simulink model "mode_lame_2019b_tentative2"  (R2020b)
settings: Solver=VariableStepAuto  StartTime=0.0  StopTime=10  RelTol=1e-3
settings Model: Creator=antoi  LastModifiedBy=antoi
settings DebuggingCC: UnderSpecifiedDimensionMsg=warning

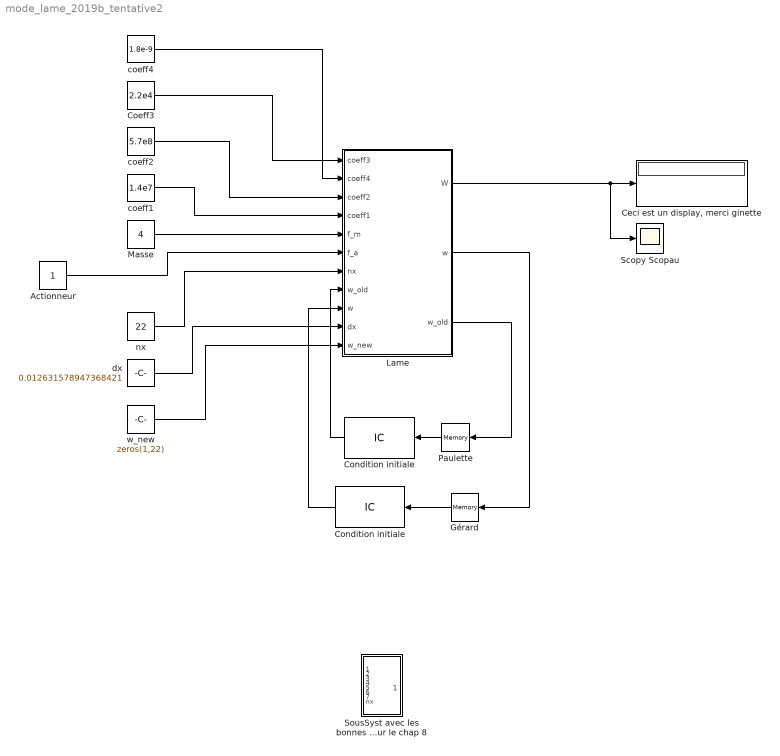
== system mode_lame_2019b_tentative2 ==
  Actionneur : Constant
  "Ceci est un display, merci ginette" : Display
  Coeff3 : Constant  Value=2.2e4
  Condition initiale : InitialCondition  Value=zeros(1,22)
  "Condition initiale " : InitialCondition  Value=zeros(1,22)
  Gérard : Memory
  Lame : MATLAB Function  TreatAsAtomicUnit=on
  Masse : Constant  Value=4
  Paulette : Memory
  Scopy Scopau : Scope
  SousSyst avec les bonnes entrées pour le chap 8 : Subsystem
  coeff1 : Constant  Value=1.4e7
  coeff2 : Constant  Value=5.7e8
  coeff4 : Constant  Value=1.8e-9
  dx : Constant  Value=0.012631578947368421
  nx : Constant  Value=22
  w_new : Constant  Value=zeros(1,22)
  wires:
  Masse/1 -> Lame/5(f_m)
  Lame/2(w) -> Gérard/1
  Lame/3(w_old) -> Paulette/1
  Gérard/1 -> Condition initiale/1
  Paulette/1 -> "Condition initiale "/1
  Lame/1(W) -> Scopy Scopau/1, "Ceci est un display, merci ginette"/1
  Coeff3/1 -> Lame/1(coeff3)
  coeff4/1 -> Lame/2(coeff4)
  nx/1 -> Lame/7(nx)
  "Condition initiale "/1 -> Lame/8("w_old ")
  Condition initiale/1 -> Lame/9("w ")
  coeff2/1 -> Lame/3(coeff2)
  dx/1 -> Lame/10(dx)
  w_new/1 -> Lame/11(w_new)
  Actionneur/1 -> Lame/6(f_a)
  coeff1/1 -> Lame/4(coeff1)

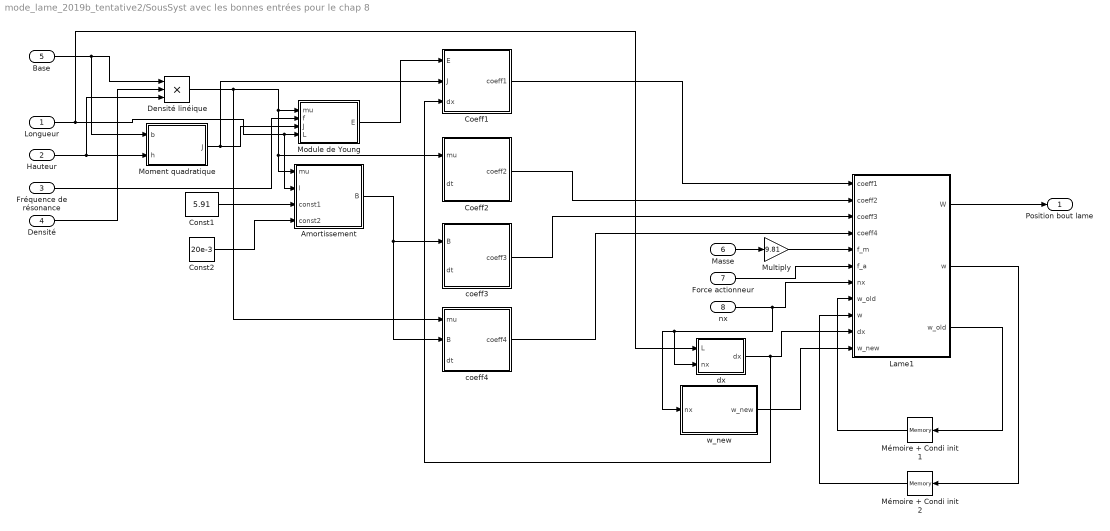
== system mode_lame_2019b_tentative2/SousSyst avec les bonnes entrées pour le chap 8 ==
  Longueur : Inport
  Hauteur : Inport  Port=2
  Fréquence de résonance : Inport  Port=3
  Densité : Inport  Port=4
  Base : Inport  Port=5
  Masse : Inport  Port=6
  Force actionneur : Inport  Port=7
  nx : Inport  Port=8
  Amortissement : MATLAB Function  TreatAsAtomicUnit=on
  Coeff1 : MATLAB Function  TreatAsAtomicUnit=on
  Coeff2 : MATLAB Function  TreatAsAtomicUnit=on
  Const1 : Constant  Value=5.91
  Const2 : Constant  Value=20e-3
  Densité linéique : Product  Inputs=3
  Lame1 : MATLAB Function  TreatAsAtomicUnit=on
  Module de Young : MATLAB Function  TreatAsAtomicUnit=on
  Moment quadratique : MATLAB Function  TreatAsAtomicUnit=on
  Multiply : Gain  Gain=9.81
  Mémoire + Condi init 1 : Memory  InitialCondition=zeros(1,22)
  Mémoire + Condi init 2 : Memory  InitialCondition=zeros(1,22)
  coeff3 : MATLAB Function  TreatAsAtomicUnit=on
  coeff4 : MATLAB Function  TreatAsAtomicUnit=on
  dx : MATLAB Function  TreatAsAtomicUnit=on
  w_new : MATLAB Function  TreatAsAtomicUnit=on
  Position bout lame : Outport
  wires:
  Lame1/3(w_old) -> Mémoire + Condi init 1/1
  Lame1/2(w) -> Mémoire + Condi init 2/1
  Mémoire + Condi init 1/1 -> Lame1/8("w_old ")
  Mémoire + Condi init 2/1 -> Lame1/9("w ")
  Lame1/1(W) -> Position bout lame/1
  Base/1 -> Moment quadratique/1(b), Densité linéique/1
  Densité/1 -> Densité linéique/2
  Hauteur/1 -> Densité linéique/3, Moment quadratique/2(h)
  Densité linéique/1 -> coeff4/1(mu), Coeff2/1(mu), Amortissement/1(mu), Module de Young/1(mu)
  Moment quadratique/1(J) -> Coeff1/2(J), Module de Young/3(J)
  Fréquence de résonance/1 -> Module de Young/2(f)
  Longueur/1 -> dx/1(L), Amortissement/2(l), Module de Young/4(L)
  Const1/1 -> Amortissement/3(const1)
  Const2/1 -> Amortissement/4(const2)
  Coeff1/1(coeff1) -> Lame1/1(coeff1)
  Coeff2/1(coeff2) -> Lame1/2(coeff2)
  coeff3/1(coeff3) -> Lame1/3(coeff3)
  coeff4/1(coeff4) -> Lame1/4(coeff4)
  Masse/1 -> Multiply/1
  Multiply/1 -> Lame1/5(f_m)
  Force actionneur/1 -> Lame1/6(f_a)
  nx/1 -> w_new/1(nx), dx/2(nx), Lame1/7(nx)
  dx/1(dx) -> Coeff1/3(dx), Lame1/10(dx)
  w_new/1(w_new) -> Lame1/11(w_new)
  Module de Young/1(E) -> Coeff1/1(E)
  Amortissement/1(B) -> coeff4/2(B), coeff3/1(B)

== matlab function mode_lame_2019b_tentative2/SousSyst avec les bonnes entrées pour le chap 8/Coeff2 ==
  data: mu input; coeff2 output; dt input
function coeff2 = fcn(mu, dt)

coeff2 = mu/(dt^2);

== matlab function mode_lame_2019b_tentative2/SousSyst avec les bonnes entrées pour le chap 8/Coeff1 ==
  data: E input; coeff1 output; J input; dx input
function coeff1 = fcn(E, J, dx)

coeff1 = (E * J)/(dx^4);

== matlab function mode_lame_2019b_tentative2/SousSyst avec les bonnes entrées pour le chap 8/dx ==
  data: L input; dx output; nx input
function dx = fcn(L, nx)

dx = L/(nx-1);

== matlab function mode_lame_2019b_tentative2/SousSyst avec les bonnes entrées pour le chap 8/w_new ==
  data: w_new output; nx input
function w_new = fcn(nx)

w_new = zeroes(1,nx);

== matlab function mode_lame_2019b_tentative2/SousSyst avec les bonnes entrées pour le chap 8/Lame1 ==
  data: coeff1 input; coeff2 input; coeff3 input; coeff4 input; f_m input; W output; f_a input; nx input; w_old input; w input; dx input; w output; w_old output; w_new input
function [W, w, w_old] = fcn(coeff1, coeff2, coeff3, coeff4, f_m, f_a, nx, w_old, w, dx, w_new) 
    
    % Vecteur position
    %w_new = zeros(1,nx); %PO y dit non non non
    
    
    % La force
    F = zeros(1, nx);
    F(11) = f_a + f_m;
    
    
%     h = plot(x, w_init, x, w_new);
%     xlabel("X [m]")
%     ylabel("Déflexion [m]")
%     ylim([-0.01,0.01])
%     grid on

    
    for i = 3:nx-2
        
        %Équation différentielle résolue par Sam
        w_new(i) = (-coeff1*(w(i+2)-4*w(i+1)+6*w(i)-4*w(i-1)+w(i-2)) - coeff2*(-2*w(i)+w_old(i)) + coeff3*w(i) + F(i)/dx)*coeff4;

        %% Conditions limites 
        w_new(1:2) =0;                 % Clampé à zero, position et dérivée nulle (le bout de la lame est fixe)

        w_new(end-1) = 2*w_new(end-2)-w_new(end-3);    % Libre au bout dérivées 2e et 3e nulles
        w_new(end) = 2*w_new(end-1)-w_new(end-2);
        
%         set(h(2), "Ydata", w_new);
%         drawnow
    end
     
    %% Préparation du prochain tour
    
    w_old = w;
    w = w_new;
    W = w(end);
end

== matlab function mode_lame_2019b_tentative2/Lame ==
  data: coeff3 input; coeff4 input; coeff2 input; coeff1 input; f_m input; W output; f_a input; nx input; w_old input; w input; dx input; w output; w_old output; w_new input
function [W, w, w_old] = fcn(coeff3, coeff4, coeff2, coeff1, f_m, f_a, nx, w_old, w, dx, w_new) 
    
    % Vecteur position
    %w_new = zeros(1,nx); %PO y dit non non non
    
    
    % La force
    F = zeros(1, nx);
    F(11) = f_a + f_m;
    
    
%     h = plot(x, w_init, x, w_new);
%     xlabel("X [m]")
%     ylabel("Déflexion [m]")
%     ylim([-0.01,0.01])
%     grid on

    
    for i = 3:nx-2
        
        %Équation différentielle résolue par Sam
        w_new(i) = (-coeff1*(w(i+2)-4*w(i+1)+6*w(i)-4*w(i-1)+w(i-2)) - coeff2*(-2*w(i)+w_old(i)) + coeff3*w(i) + F(i)/dx)*coeff4;

        %% Conditions limites 
        w_new(1:2) =0;                 % Clampé à zero, position et dérivée nulle (le bout de la lame est fixe)

        w_new(end-1) = 2*w_new(end-2)-w_new(end-3);    % Libre au bout dérivées 2e et 3e nulles
        w_new(end) = 2*w_new(end-1)-w_new(end-2);
        
%         set(h(2), "Ydata", w_new);
%         drawnow
    end
     
    %% Préparation du prochain tour
    
    w_old = w;
    w = w_new;
    W = w(end);
end

== matlab function mode_lame_2019b_tentative2/SousSyst avec les bonnes entrées pour le chap 8/Moment quadratique ==
  data: b input; J output; h input
function J = fcn(b, h)

J = b*h^3/12;

== matlab function mode_lame_2019b_tentative2/SousSyst avec les bonnes entrées pour le chap 8/Module de Young ==
  data: mu input; E output; f input; J input; L input
function E = fcn(mu, f, J, L)

E = (mu*(2*pi*f)^2/J)*(L/1.875)^4;

== matlab function mode_lame_2019b_tentative2/SousSyst avec les bonnes entrées pour le chap 8/Amortissement ==
  data: mu input; B output; l input; const1 input; const2 input
function B = fcn(mu, l, const1, const2)

B = const1 * (mu * l + const2);

== matlab function mode_lame_2019b_tentative2/SousSyst avec les bonnes entrées pour le chap 8/coeff4 ==
  data: mu input; coeff4 output; B input; dt input
function coeff4 = fcn(mu, B, dt)

coeff4 = ((mu/dt^2)+(B/dt))^(-1);

== matlab function mode_lame_2019b_tentative2/SousSyst avec les bonnes entrées pour le chap 8/coeff3 ==
  data: B input; coeff3 output; dt input
function coeff3 = fcn(B, dt)

coeff3 = B/dt;
